simulink model "resp_sostenidav2015b"  (R2015b)
settings: Solver=ode4  SolverMode=SingleTasking  StartTime=0.0  StopTime=6.0  FixedStep=0.02  RelTol=1e-3
undefined symbols (not defined in the file): de_pos_disc, Kc, nu_pos_disc
settings Model: Creator=growin  LastModifiedBy=sersanc8
settings DataIOCC: LimitDataPoints=off
settings DebuggingCC: AllowSymbolicDim=on  SFUnexpectedBacktrackingDiag=error  SFNoUnconditionalDefaultTransitionDiag=error
settings ModelReferenceCC: PropagateSignalLabelsOutOfModel=on
settings GRTTargetCC: TargetLangStandard=C99 (ISO)
settings ConfigComp: CovMetricSettings=dwe  CovHtmlReporting=off  CovSaveCumulativeToWorkspaceVar=off  CovSaveSingleToWorkspaceVar=off  CovModelRefEnable=Off  CovExternalEMLEnable=on

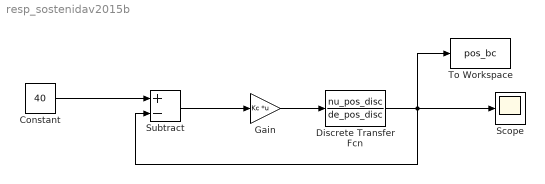
== system resp_sostenidav2015b ==
  Constant : Constant  Value=40
  Discrete Transfer Fcn : DiscreteTransferFcn  Numerator=nu_pos_disc  Denominator=de_pos_disc  SampleTime=0.02
  Gain : Gain  Gain=Kc  Multiplication=Matrix(K*u)
  Scope : Scope
  Subtract : Sum  Inputs=+-
  To Workspace : ToWorkspace  VariableName=pos_bc  SampleTime=-1
  wires:
  Constant/1 -> Subtract/1
  Subtract/1 -> Gain/1
  Gain/1 -> Discrete Transfer Fcn/1
  Discrete Transfer Fcn/1 -> Subtract/2, Scope/1, To Workspace/1
